simulink model "pathPlanningVPP"  (R2023a)
settings: Solver=VariableStepAuto  StartTime=0.0  StopTime=0.1  RelTol=1e-3
values from neighbouring files (symbols this model uses):
  egoInitialPose = [7,3.1,0]    [PlanParallelParkingPathUsingMultistageNonlinearMPC1.m]
  egoTargetPose = [-1.4,0,0]    [PlanParallelParkingPathUsingMultistageNonlinearMPC1.m]
  Ts = 1    [PlanParallelParkingPathUsingMultistageNonlinearMPC1.m]
libraries: mpcadaslib x1
settings Model: Creator=The MathWorks, Inc.  LastModifiedBy=The MathWorks, Inc.
settings SolverCC: MaxZcPerStep=1
settings OptimizationCC: ReuseModelBlockBuffer=off

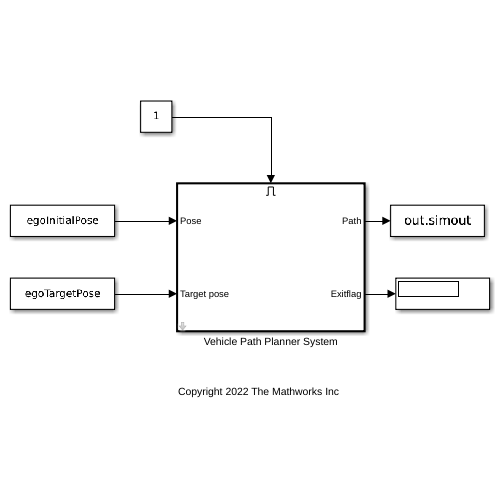
[thumbnail: Simulink's stored preview of the top-level diagram]
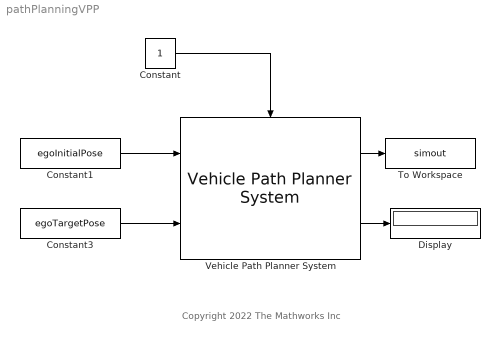
== system pathPlanningVPP ==
  note: Copyright 2022 The Mathworks Inc
  Constant : Constant
  Constant1 : Constant  Value=egoInitialPose  VectorParams1D=off
  Constant3 : Constant  Value=egoTargetPose  VectorParams1D=off
  Display : Display
  To Workspace : ToWorkspace  VariableName=simout  SampleTime=-1
  Vehicle Path Planner System : mpcadaslib/Vehicle Path Planner System  egoLength=4.7  egoWidth=1.8  wheelbase=2.8  dist2Center=1.4  numObs=numObs  obsMat=obsMat  obs_ext=off  minDist=d_safe  Ts=Ts  pPlanning=p  v_range=v_range  v_ext=off  steer_range=steer_range  steer_ext=off  suboptimal=off  maxiter=200  output_exitflag=on
      settings: LibrarySourceBlock=mpclib/Automated Driving/Vehicle Path Planner System
  wires:
  Constant/1 -> Vehicle Path Planner System/Enable
  Constant3/1 -> Vehicle Path Planner System/2
  Constant1/1 -> Vehicle Path Planner System/1
  Vehicle Path Planner System/2 -> Display/1
  Vehicle Path Planner System/1 -> To Workspace/1
